simulink model "d2_model"  (R2021b)
settings: Solver=VariableStepAuto  StartTime=0.0  StopTime=40  RelTol=1e-3
values from neighbouring files (symbols this model uses):
  A = [0 1 0 0; -K_m/M 0 K_m/M 0; 0 0 0 1; K_m/M 0 -K_m/M 0]    [d2.m]
  Ao = [Ai zeros(3, 3); zeros(3, 3) Ai]    [d2.m]
  At = [A B*Co; zeros(6, 4) Ao]    [d2.m]
  B = [0 0; 1/M 0; 0 0; 0 1/M]    [d2.m]
  Bo = [Bi zeros(3, 1); zeros(3, 1) Bi]    [d2.m]
  Bt = [B zeros(4, 2); zeros(6, 2) Bo]    [d2.m]
  C = [1 0 0 0; 0 0 1 0]    [d2.m]
  Co = [Ci zeros(1, 3); zeros(1, 3) Ci]    [d2.m]
  Ct = [C zeros(2, 6)]    [d2.m]
  D = [0 0; 0 0]    [d2.m]
  Do = zeros(2, 2)    [d2.m]
  Ft = -K    [d2.m]
  Kt = H'    [d2.m]
settings Model: Creator=Murillo  LastModifiedBy=Murillo

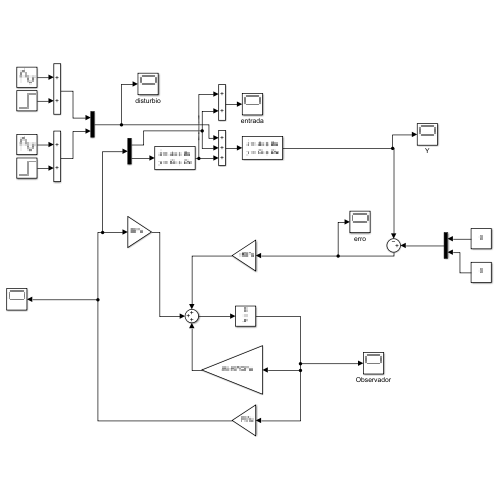
[thumbnail: Simulink's stored preview of the top-level diagram]
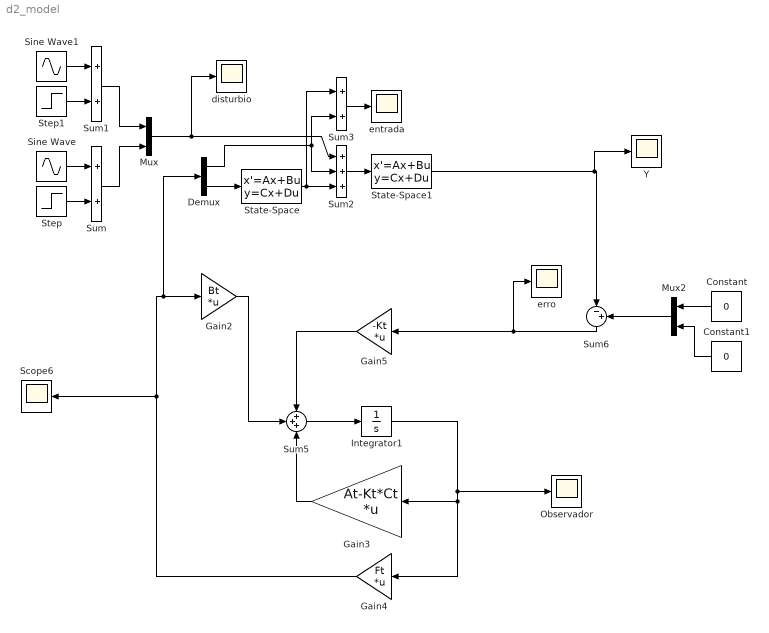
== system d2_model ==
  Constant : Constant  Value=0
  Constant1 : Constant  Value=0
  Demux : Demux  Outputs=2
  Gain2 : Gain  Gain=Bt  Multiplication=Matrix(K*u)
  Gain3 : Gain  Gain=At-Kt*Ct  Multiplication=Matrix(K*u)
  Gain4 : Gain  Gain=Ft  Multiplication=Matrix(K*u)
  Gain5 : Gain  Gain=-Kt  Multiplication=Matrix(K*u)
  Integrator1 : Integrator
  Mux : Mux  Inputs=2
  Mux2 : Mux  Inputs=2
  Observador : Scope
  Scope6 : Scope
  Sine Wave : Sin  Amplitude=0.5  Frequency=0.5  Phase=10  SampleTime=0
  Sine Wave1 : Sin  Frequency=0.5  Phase=pi/4  SampleTime=0
  State-Space : StateSpace  A=Ao  B=Bo  C=Co  D=Do  InitialCondition=0
  State-Space1 : StateSpace  A=A  B=B  C=C  D=D  InitialCondition=0
  Step : Step  SampleTime=0
  Step1 : Step  SampleTime=0
  Sum : Sum
  Sum1 : Sum
  Sum2 : Sum  Inputs=+++
  Sum3 : Sum
  Sum5 : Sum  Inputs=+++
  Sum6 : Sum  Inputs=|-+
  Y : Scope
  disturbio : Scope
  entrada : Scope
  erro : Scope
  wires:
  Step/1 -> Sum/2
  Sine Wave/1 -> Sum/1
  Sine Wave1/1 -> Sum1/1
  Step1/1 -> Sum1/2
  Sum1/1 -> Mux/1
  Sum/1 -> Mux/2
  State-Space/1 -> Sum3/1, Sum2/3
  Demux/2 -> State-Space/1
  Demux/1 -> Sum2/2, Sum3/2
  Mux/1 -> Sum2/1, disturbio/1
  Sum2/1 -> State-Space1/1
  Sum3/1 -> entrada/1
  Constant1/1 -> Mux2/2
  Gain3/1 -> Sum5/3
  Integrator1/1 -> Gain4/1, Gain3/1, Observador/1
  Mux2/1 -> Sum6/2
  Gain5/1 -> Sum5/1
  Gain2/1 -> Sum5/2
  Constant/1 -> Mux2/1
  Sum6/1 -> erro/1, Gain5/1
  Gain4/1 -> Gain2/1, Demux/1, Scope6/1
  Sum5/1 -> Integrator1/1
  State-Space1/1 -> Y/1, Sum6/1
